simulink model "compensacion_digital_integrador"  (R2014b)
settings: Solver=ode45  StartTime=0.0  StopTime=4  RelTol=1e-3
settings Model: Creator=Javi  LastModifiedBy=Javi

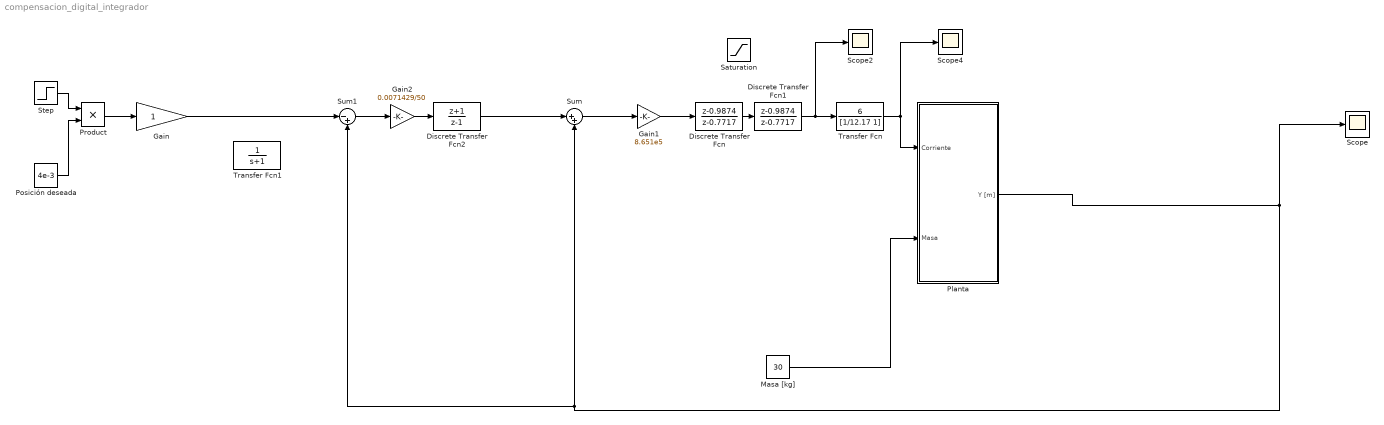
== system compensacion_digital_integrador ==
  Discrete Transfer Fcn : DiscreteTransferFcn  Numerator=[1 -0.9874]  Denominator=[1 -0.7717]  SampleTime=1/3.5e3
  Discrete Transfer Fcn1 : DiscreteTransferFcn  Numerator=[1 -0.9874]  Denominator=[1 -0.7717]
  Discrete Transfer Fcn2 : DiscreteTransferFcn  Numerator=[1 1]  Denominator=[1 -1]  SampleTime=1/3.5e3
  Gain : Gain
  Gain1 : Gain  Gain=8.651e5
  Gain2 : Gain  Gain=0.0071429/50
  "Masa [kg] " : Constant  Value=30
  "Planta " : Subsystem
  Posición deseada : Constant  Value=4e-3
  Product : Product
  Saturation : Saturate  UpperLimit=5  LowerLimit=-inf
  Scope : Scope
      settings: TimeRange=4  YMin=0  YMax=0.014
  Scope2 : Scope
      settings: TimeRange=0.1399527394936923  YMin=-30.18303415559998  YMax=56.43935634467678  SaveName=ScopeData2
  Scope4 : Scope
      settings: TimeRange=0.005185185185185187  YMin=-3500000  YMax=500000  SaveName=ScopeData4
  Step : Step  Time=0.01  SampleTime=0
  Sum : Sum  Inputs=|++
  Sum1 : Sum  Inputs=|-+
  Transfer Fcn : TransferFcn  Numerator=[6]  Denominator=[1/12.17 1]
  Transfer Fcn1 : TransferFcn  Denominator=[1 1]
  wires:
  "Masa [kg] "/1 -> "Planta "/2("Masa ")
  "Planta "/1(Y [m]) -> Scope/1, Sum1/2, Sum/2
  Transfer Fcn/1 -> "Planta "/1(Corriente), Scope4/1
  Discrete Transfer Fcn1/1 -> Scope2/1, Transfer Fcn/1
  Step/1 -> Product/1
  Posición deseada/1 -> Product/2
  Product/1 -> Gain/1
  Gain1/1 -> Discrete Transfer Fcn/1
  Sum/1 -> Gain1/1
  Discrete Transfer Fcn/1 -> Discrete Transfer Fcn1/1
  Discrete Transfer Fcn2/1 -> Sum/1
  Sum1/1 -> Gain2/1
  Gain2/1 -> Discrete Transfer Fcn2/1
  Gain/1 -> Sum1/1

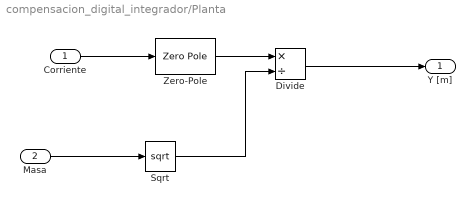
== system compensacion_digital_integrador/Planta  ==
  Corriente : Inport
  "Masa " : Inport  Port=2
  Divide : Product  Inputs=*/
  Sqrt : Sqrt  SaturateOnIntegerOverflow=on
  Zero-Pole : ZeroPole  Zeros=[]  Poles=[70 -70]  Gain=-6.58
  Y [m] : Outport
  wires:
  Divide/1 -> Y [m]/1
  Corriente/1 -> Zero-Pole/1
  Zero-Pole/1 -> Divide/1
  "Masa "/1 -> Sqrt/1
  Sqrt/1 -> Divide/2
